simulink library "HeightCalcLib"  (R2018b)
settings: Solver=VariableStepAuto  StartTime=0.0  StopTime=10.0  RelTol=1e-3
settings Model: Creator=sn2xws  LastModifiedBy=sn2xws

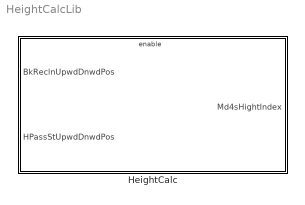
== system HeightCalcLib ==
  HeightCalc : Subsystem

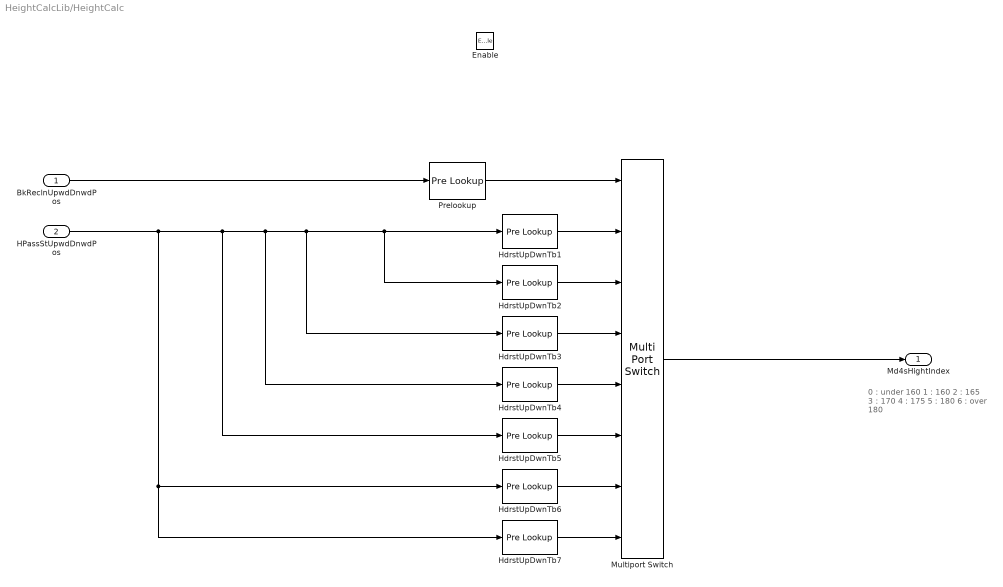
== system HeightCalcLib/HeightCalc ==
  note: 0：under 160
      | 1：160
      | 2：165
      | 3：170
      | 4：175
      | 5：180
      | 6：over 180
  BkReclnUpwdDnwdPos : Inport
  HPassStUpwdDnwdPos : Inport  Port=2
  Enable : EnablePort
  HdrstUpDwnTb1 : PreLookup  BreakpointsData=KeSMSw4SAdpnHdrstUpwdDnwdPos1_Val  OutputSelection=Index only  IndexDataTypeStr=uint8
  HdrstUpDwnTb2 : PreLookup  BreakpointsData=KeSMSw4SAdpnHdrstUpwdDnwdPos2_Val  OutputSelection=Index only  IndexDataTypeStr=uint8
  HdrstUpDwnTb3 : PreLookup  BreakpointsData=KeSMSw4SAdpnHdrstUpwdDnwdPos3_Val  OutputSelection=Index only  IndexDataTypeStr=uint8
  HdrstUpDwnTb4 : PreLookup  BreakpointsData=KeSMSw4SAdpnHdrstUpwdDnwdPos4_Val  OutputSelection=Index only  IndexDataTypeStr=uint8
  HdrstUpDwnTb5 : PreLookup  BreakpointsData=KeSMSw4SAdpnHdrstUpwdDnwdPos5_Val  OutputSelection=Index only  IndexDataTypeStr=uint8
  HdrstUpDwnTb6 : PreLookup  BreakpointsData=KeSMSw4SAdpnHdrstUpwdDnwdPos6_Val  OutputSelection=Index only  IndexDataTypeStr=uint8
  HdrstUpDwnTb7 : PreLookup  BreakpointsData=KeSMSw4SAdpnHdrstUpwdDnwdPos7_Val  OutputSelection=Index only  IndexDataTypeStr=uint8
  Multiport Switch : MultiPortSwitch  DataPortOrder=Zero-based contiguous  Inputs=7  DiagnosticForDefault=None  zeroidx=on
  Prelookup : PreLookup  BreakpointsData=KeSMSw4SAdpnReclnUpwdDnwdPos_Val  OutputSelection=Index only  IndexDataTypeStr=uint8
  Md4sHightIndex : Outport
  wires:
  HdrstUpDwnTb6/1 -> Multiport Switch/7
  HPassStUpwdDnwdPos/1 -> HdrstUpDwnTb7/1, HdrstUpDwnTb6/1, HdrstUpDwnTb5/1, HdrstUpDwnTb4/1, HdrstUpDwnTb3/1, HdrstUpDwnTb2/1, HdrstUpDwnTb1/1
  HdrstUpDwnTb2/1 -> Multiport Switch/3
  HdrstUpDwnTb5/1 -> Multiport Switch/6
  HdrstUpDwnTb4/1 -> Multiport Switch/5
  Multiport Switch/1 -> Md4sHightIndex/1
  HdrstUpDwnTb1/1 -> Multiport Switch/2
  BkReclnUpwdDnwdPos/1 -> Prelookup/1
  HdrstUpDwnTb7/1 -> Multiport Switch/8
  Prelookup/1 -> Multiport Switch/1
  HdrstUpDwnTb3/1 -> Multiport Switch/4
